simulink model "PubIfFusionRFM_MDL"  (R2020b)
settings: Solver=FixedStepAuto  StartTime=0.0  StopTime=Inf  RelTol=1e-3
PostLoadFcn:
  | if any(exist('dsrtsu_mdlpostloadfcn', 'file') ~= 0), dsrtsu_mdlpostloadfcn('Execute', bdroot); end
InitFcn:
  | , if any(exist('dsmpb_private', 'file') ~= 0), dsmpb_private('dsmpb_mdlclblib', 'Init', bdroot); end,
model workspace (MAT data in the model file):
  EQ4COM_BrkPedalSts = Simulink.Signal
  EQ4COM_BrkPedalSts.DataType = 'auto'
  EQ4COM_BrkPedalSts.Dimensions = -1
  EQ4COM_BrkPedalSts.DimensionsMode = 'auto'
  EQ4COM_BrkPedalSts.Complexity = 'auto'
  EQ4COM_BrkPedalSts.SampleTime = -1
  EQ4COM_BrkPedalSts.SamplingMode = 'auto'
  EQ4COM_ESP_MasterCylBrkPress = Simulink.Signal
  EQ4COM_ESP_MasterCylBrkPress.DataType = 'auto'
  EQ4COM_ESP_MasterCylBrkPress.Dimensions = -1
  EQ4COM_ESP_MasterCylBrkPress.DimensionsMode = 'auto'
  EQ4COM_ESP_MasterCylBrkPress.Complexity = 'auto'
  EQ4COM_ESP_MasterCylBrkPress.SampleTime = -1
  EQ4COM_ESP_MasterCylBrkPress.SamplingMode = 'auto'
  EQ4COM_SteerWheelAng = Simulink.Signal
  EQ4COM_SteerWheelAng.DataType = 'auto'
  EQ4COM_SteerWheelAng.Dimensions = -1
  EQ4COM_SteerWheelAng.DimensionsMode = 'auto'
  EQ4COM_SteerWheelAng.Complexity = 'auto'
  EQ4COM_SteerWheelAng.SampleTime = -1
  EQ4COM_SteerWheelAng.SamplingMode = 'auto'
  EQ4COM_SteerWheelAngSign = Simulink.Signal
  EQ4COM_SteerWheelAngSign.DataType = 'auto'
  EQ4COM_SteerWheelAngSign.Dimensions = -1
  EQ4COM_SteerWheelAngSign.DimensionsMode = 'auto'
  EQ4COM_SteerWheelAngSign.Complexity = 'auto'
  EQ4COM_SteerWheelAngSign.SampleTime = -1
  EQ4COM_SteerWheelAngSign.SamplingMode = 'auto'
  EQ4COM_VehLatAccel = Simulink.Signal
  EQ4COM_VehLatAccel.DataType = 'auto'
  EQ4COM_VehLatAccel.Dimensions = -1
  EQ4COM_VehLatAccel.DimensionsMode = 'auto'
  EQ4COM_VehLatAccel.Complexity = 'auto'
  EQ4COM_VehLatAccel.SampleTime = -1
  EQ4COM_VehLatAccel.SamplingMode = 'auto'
  EQ4COM_VehLgtAccel = Simulink.Signal
  EQ4COM_VehLgtAccel.DataType = 'auto'
  EQ4COM_VehLgtAccel.Dimensions = -1
  EQ4COM_VehLgtAccel.DimensionsMode = 'auto'
  EQ4COM_VehLgtAccel.Complexity = 'auto'
  EQ4COM_VehLgtAccel.SampleTime = -1
  EQ4COM_VehLgtAccel.SamplingMode = 'auto'
  EQ4COM_VehSpd = Simulink.Signal
  EQ4COM_VehSpd.DataType = 'auto'
  EQ4COM_VehSpd.Dimensions = -1
  EQ4COM_VehSpd.DimensionsMode = 'auto'
  EQ4COM_VehSpd.Complexity = 'auto'
  EQ4COM_VehSpd.SampleTime = -1
  EQ4COM_VehSpd.SamplingMode = 'auto'
  EQ4COM_VehYawRate = Simulink.Signal
  EQ4COM_VehYawRate.DataType = 'auto'
  EQ4COM_VehYawRate.Dimensions = -1
  EQ4COM_VehYawRate.DimensionsMode = 'auto'
  EQ4COM_VehYawRate.Complexity = 'auto'
  EQ4COM_VehYawRate.SampleTime = -1
  EQ4COM_VehYawRate.SamplingMode = 'auto'
PreSaveFcn:
  | , if any(exist('dsmpb_private', 'file') ~= 0), dsmpb_private('dsmpb_mdlclblib', 'PreSave', bdroot); end,
CloseFcn:
  | , if any(exist('dsmpb_private', 'file') ~= 0), dsmpb_private('dsmpb_mdlclblib', 'Close', bdroot); end,
settings Model: DataDictionary=HWA_DDs.sldd  RTICANMMDATA=struct('GeneralSetupData',struct('modelroot','C:\Users\GW00133806\Desktop\ADAS_Store\Project\V61_Autobox_Noa\Fusion\fusRoad','generalsettings',struct('filesettings',struct('destfolder',struct('Name','RTICANMM_FILES','Check',1),'buildfolder',struct('Name','.','Check',1),'AbsDestfolder',struct('Name','C:\Users\GW00133806\Desktop\ADAS_Store\Project\V61_Autobox_Noa\Fusion\fusRoad\RTICANMM_FILES'),'AbsBuildfolder',struct('Name','C:\Users\GW00133806\Desktop\ADAS_Store\Project\V61_Autobox_Noa\Fusion\fusRoad'))),'options',struct('addpaths',1,'rmpaths',1,'addtrcexclusion',false,'cannavigator',struct('checkmonitoring',0),'show_usrtrc',0,'use_usrtrc',0),'advanced',struct('options',ones(1,100)),'MPSetup',{{}},'RTI',struct('Type','DSRT','Ver','4.2','Date','02-Nov-2019'),'modelname','PubIfFusionRFM_MDL','block','PubIfFusionRFM_MDL'))  DSRTSU_INTERNAL_RTIFPGA=150  Creator=GW00180895  LastModifiedBy=GW00133806
settings OptimizationCC: BlockReduction=off  ConditionallyExecuteInputs=off  OptimizeBlockIOStorage=off  BufferReuse=off
settings DebuggingCC: TasksWithSamePriorityMsg=none
settings HardwareCC: ProdBitPerPointer=32  ProdBitPerSizeT=32  ProdBitPerPtrDiffT=32  ProdLargestAtomicInteger=Integer  ProdWordSize=32  ProdHWDeviceType=Custom Processor->Custom
settings ModelReferenceCC: EnableParallelModelReferenceBuilds=on  ModelReferenceNumInstancesAllowed=Single  SupportModelReferenceSimTargetCustomCode=on
settings SFSimCC: SimParseCustomCode=off  MATLABDynamicMemAlloc=off
settings SFSimCC: SimUserSources=|
  | FusionApi.c
  | HWAapi.c
  | HWA_R.c
  | HWAafRoadArithm.c
  | HWABoundary.c
  | HWABoundaryLinePredicted.c
  | HWALineFusion.c
  | HWAObejctManage.c
  | HWARoadLayout.c
  | HWARoadPreprocess.c
  | HWARoadSceneRecognition.c
  | HWASpeedLimit.c
  | HWAOutputSendCallback.c
settings SFSimCC: SimUserIncludeDirs=|
  | .\src\HWA_Road\include
  | .\src\HWA_Road\include\HWAMsg
  | .\src\HWA_Road\include\HWAPack
  | .\src\HWA_Road\include\HWAApi
  | .\src\HWA_Road\source
  | .\src\HWA_Road\source\Road
  | .\src\HWA_Road_Api
  | .\src\HWA_Road_Api\autosar_swc_infofusion_autosar_rtw
  | .\src
settings RTWCC: Description=dSPACE Run-Time Target (for VEOS on Windows and ConfigurationDesk)  SystemTargetFile=dsrt.tlc  GenCodeOnly=on  MakeCommand=make_dsrt  TemplateMakefile=dsrt_default_tmf  RTWVerbose=off  RTWUseSimCustomCode=on
settings RTWCC: CustomInclude=|
  | .\src\HWA_Road\include
  | .\src\HWA_Road\include\HWAMsg
  | .\src\HWA_Road\include\HWAPack
  | .\src\HWA_Road\include\HWAApi
  | .\src\HWA_Road\source
  | .\src\HWA_Road\source\Road
  | .\src\HWA_Road_Api
  | .\src\HWA_Road_Api\autosar_swc_infofusion_autosar_rtw
  | .\src
settings RTWCC: CustomSource=|
  | FusionApi.c
  | HWAapi.c
  | HWA_R.c
  | HWAafRoadArithm.c
  | HWABoundary.c
  | HWABoundaryLinePredicted.c
  | HWALineFusion.c
  | HWAObejctManage.c
  | HWARoadLayout.c
  | HWARoadPreprocess.c
  | HWARoadSceneRecognition.c
  | HWASpeedLimit.c
  | HWAOutputSendCallback.c
settings STFCustomTargetCC: TargetLangStandard=C99 (ISO)  ParMdlRefBuildCompliant=on  ConcurrentExecutionCompliant=off  CPPClassGenCompliant=off  GRTInterface=off  SystemTargetFile=dsrt.tlc
settings GRTTargetCC: CompOptLevelCompliant=off  ConcurrentExecutionCompliant=off  CombineOutputUpdateFcns=off  MatFileLogging=off  CPPClassGenCompliant=off  UseToolchainInfoCompliant=off

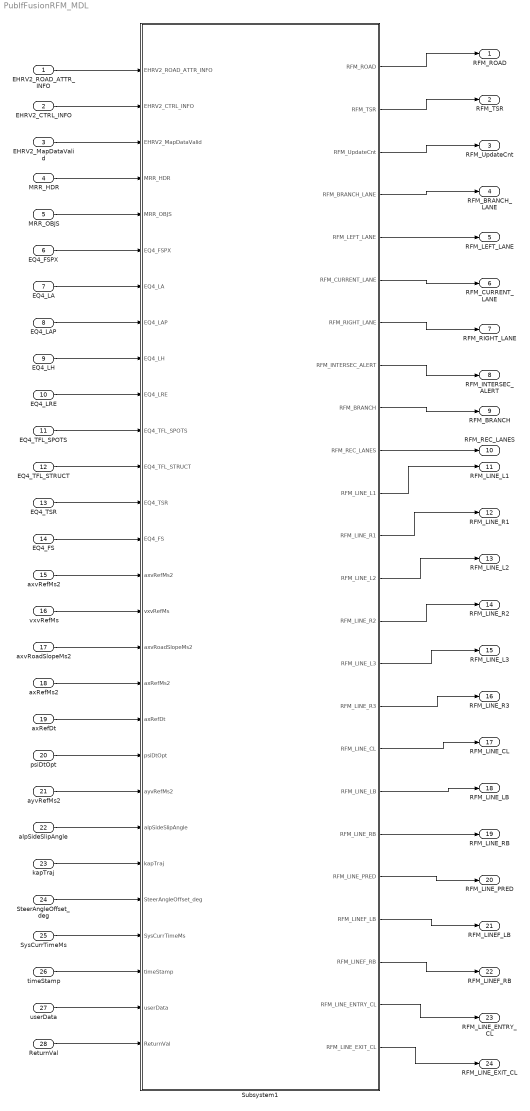
== system PubIfFusionRFM_MDL ==
  EHRV2_ROAD_ATTR_INFO : Inport  OutDataTypeStr=Bus: EHRV2_ROAD_ATTR_INFO_BUS  PortDimensions=1  BusOutputAsStruct=on
  EHRV2_CTRL_INFO : Inport  Port=2  OutDataTypeStr=Bus: EHRV2_CTRL_INFO_BUS  PortDimensions=1  BusOutputAsStruct=on
  EHRV2_MapDataValid : Inport  Port=3  OutDataTypeStr=uint8  PortDimensions=1  BusOutputAsStruct=on
  MRR_HDR : Inport  Port=4  OutDataTypeStr=Bus: MRR_HDR_BUS  PortDimensions=1  BusOutputAsStruct=on
  MRR_OBJS : Inport  Port=5  OutDataTypeStr=Bus: MRR_OBJ_BUS  PortDimensions=32  BusOutputAsStruct=on
  EQ4_FSPX : Inport  Port=6  OutDataTypeStr=Bus: EQ4_FSPX_BUS  PortDimensions=1  BusOutputAsStruct=on
  EQ4_LA : Inport  Port=7  OutDataTypeStr=Bus: EQ4_LA_BUS  PortDimensions=1  BusOutputAsStruct=on
  EQ4_LAP : Inport  Port=8  OutDataTypeStr=Bus: EQ4_LAP_BUS  PortDimensions=1  BusOutputAsStruct=on
  EQ4_LH : Inport  Port=9  OutDataTypeStr=Bus: EQ4_LH_BUS  PortDimensions=1  BusOutputAsStruct=on
  EQ4_LRE : Inport  Port=10  OutDataTypeStr=Bus: EQ4_LRE_BUS  PortDimensions=1  BusOutputAsStruct=on
  EQ4_TFL_SPOTS : Inport  Port=11  OutDataTypeStr=Bus: EQ4_TFL_SPOTS_BUS  PortDimensions=1  BusOutputAsStruct=on
  EQ4_TFL_STRUCT : Inport  Port=12  OutDataTypeStr=Bus: EQ4_TFL_STRUCT_BUS  PortDimensions=1  BusOutputAsStruct=on
  EQ4_TSR : Inport  Port=13  OutDataTypeStr=Bus: EQ4_TSR_BUS  PortDimensions=1  BusOutputAsStruct=on
  EQ4_FS : Inport  Port=14  OutDataTypeStr=Bus: EQ4_FS_BUS  PortDimensions=1  BusOutputAsStruct=on
  axvRefMs2 : Inport  Port=15  OutDataTypeStr=single  PortDimensions=1  BusOutputAsStruct=on
  vxvRefMs : Inport  Port=16  OutDataTypeStr=single  PortDimensions=1  BusOutputAsStruct=on
  axvRoadSlopeMs2 : Inport  Port=17  OutDataTypeStr=single  PortDimensions=1  BusOutputAsStruct=on
  axRefMs2 : Inport  Port=18  OutDataTypeStr=single  PortDimensions=1  BusOutputAsStruct=on
  axRefDt : Inport  Port=19  OutDataTypeStr=single  PortDimensions=1  BusOutputAsStruct=on
  psiDtOpt : Inport  Port=20  OutDataTypeStr=single  PortDimensions=1  BusOutputAsStruct=on
  ayvRefMs2 : Inport  Port=21  OutDataTypeStr=single  PortDimensions=1  BusOutputAsStruct=on
  alpSideSlipAngle : Inport  Port=22  OutDataTypeStr=single  PortDimensions=1  BusOutputAsStruct=on
  kapTraj : Inport  Port=23  OutDataTypeStr=single  PortDimensions=1  BusOutputAsStruct=on
  SteerAngleOffset_deg : Inport  Port=24  OutDataTypeStr=single  PortDimensions=1  BusOutputAsStruct=on
  SysCurrTimeMs : Inport  Port=25  OutDataTypeStr=uint32  PortDimensions=1  BusOutputAsStruct=on
  timeStamp : Inport  Port=26  OutDataTypeStr=Bus: StbM_TimeStampExtendedType  PortDimensions=1  BusOutputAsStruct=on
  userData : Inport  Port=27  OutDataTypeStr=Bus: StbM_UserDataType  PortDimensions=1  BusOutputAsStruct=on
  ReturnVal : Inport  Port=28  OutDataTypeStr=uint8  PortDimensions=1  BusOutputAsStruct=on
  Subsystem1 : Subsystem
  RFM_ROAD : Outport  OutDataTypeStr=Bus: RFM_ROAD_BUS  BusOutputAsStruct=on
  RFM_TSR : Outport  Port=2  OutDataTypeStr=Bus: RFM_TSR_BUS  PortDimensions=1  BusOutputAsStruct=on
  RFM_UpdateCnt : Outport  Port=3  OutDataTypeStr=uint32  PortDimensions=1  BusOutputAsStruct=on
  RFM_BRANCH_LANE : Outport  Port=4  OutDataTypeStr=Bus: RFM_LANE_BUS  PortDimensions=1  BusOutputAsStruct=on
  RFM_LEFT_LANE : Outport  Port=5  OutDataTypeStr=Bus: RFM_LANE_BUS  PortDimensions=1  BusOutputAsStruct=on
  RFM_CURRENT_LANE : Outport  Port=6  OutDataTypeStr=Bus: RFM_LANE_BUS  PortDimensions=1  BusOutputAsStruct=on
  RFM_RIGHT_LANE : Outport  Port=7  OutDataTypeStr=Bus: RFM_LANE_BUS  PortDimensions=1  BusOutputAsStruct=on
  RFM_INTERSEC_ALERT : Outport  Port=8  OutDataTypeStr=Bus: RFM_INTERSEC_ALERT_BUS  PortDimensions=1  BusOutputAsStruct=on
  RFM_BRANCH : Outport  Port=9  OutDataTypeStr=Bus: RFM_BRANCH_BUS  PortDimensions=1  BusOutputAsStruct=on
  RFM_REC_LANES : Outport  Port=10  OutDataTypeStr=Bus: RFM_REC_LANES_BUS  PortDimensions=1  BusOutputAsStruct=on
  RFM_LINE_L1 : Outport  Port=11  OutDataTypeStr=Bus: RFM_LINE_BUS  PortDimensions=1  BusOutputAsStruct=on
  RFM_LINE_R1 : Outport  Port=12  OutDataTypeStr=Bus: RFM_LINE_BUS  PortDimensions=1  BusOutputAsStruct=on
  RFM_LINE_L2 : Outport  Port=13  OutDataTypeStr=Bus: RFM_LINE_BUS  PortDimensions=1  BusOutputAsStruct=on
  RFM_LINE_R2 : Outport  Port=14  OutDataTypeStr=Bus: RFM_LINE_BUS  PortDimensions=1  BusOutputAsStruct=on
  RFM_LINE_L3 : Outport  Port=15  OutDataTypeStr=Bus: RFM_LINE_BUS  PortDimensions=1  BusOutputAsStruct=on
  RFM_LINE_R3 : Outport  Port=16  OutDataTypeStr=Bus: RFM_LINE_BUS  PortDimensions=1  BusOutputAsStruct=on
  RFM_LINE_CL : Outport  Port=17  OutDataTypeStr=Bus: RFM_LINE_BUS  PortDimensions=1  BusOutputAsStruct=on
  RFM_LINE_LB : Outport  Port=18  OutDataTypeStr=Bus: RFM_LINE_BUS  PortDimensions=1  BusOutputAsStruct=on
  RFM_LINE_RB : Outport  Port=19  OutDataTypeStr=Bus: RFM_LINE_BUS  PortDimensions=1  BusOutputAsStruct=on
  RFM_LINE_PRED : Outport  Port=20  OutDataTypeStr=Bus: RFM_LINE_BUS  PortDimensions=1  BusOutputAsStruct=on
  RFM_LINEF_LB : Outport  Port=21  OutDataTypeStr=Bus: RFM_LINE_BUS  PortDimensions=1  BusOutputAsStruct=on
  RFM_LINEF_RB : Outport  Port=22  OutDataTypeStr=Bus: RFM_LINE_BUS  PortDimensions=1  BusOutputAsStruct=on
  RFM_LINE_ENTRY_CL : Outport  Port=23  OutDataTypeStr=Bus: RFM_LINE_BUS  PortDimensions=1  BusOutputAsStruct=on
  RFM_LINE_EXIT_CL : Outport  Port=24  OutDataTypeStr=Bus: RFM_LINE_BUS  PortDimensions=1  BusOutputAsStruct=on
  wires:
  EHRV2_ROAD_ATTR_INFO/1 -> Subsystem1/1(EHRV2_ROAD_ATTR_INFO)
  EHRV2_CTRL_INFO/1 -> Subsystem1/2(EHRV2_CTRL_INFO)
  EHRV2_MapDataValid/1 -> Subsystem1/3(EHRV2_MapDataValid)
  MRR_HDR/1 -> Subsystem1/4(MRR_HDR)
  MRR_OBJS/1 -> Subsystem1/5(MRR_OBJS)
  EQ4_FSPX/1 -> Subsystem1/6(EQ4_FSPX)
  EQ4_LA/1 -> Subsystem1/7(EQ4_LA)
  EQ4_LAP/1 -> Subsystem1/8(EQ4_LAP)
  EQ4_LH/1 -> Subsystem1/9(EQ4_LH)
  EQ4_LRE/1 -> Subsystem1/10(EQ4_LRE)
  EQ4_TFL_SPOTS/1 -> Subsystem1/11(EQ4_TFL_SPOTS)
  EQ4_TFL_STRUCT/1 -> Subsystem1/12(EQ4_TFL_STRUCT)
  EQ4_TSR/1 -> Subsystem1/13(EQ4_TSR)
  EQ4_FS/1 -> Subsystem1/14(EQ4_FS)
  axvRefMs2/1 -> Subsystem1/15(axvRefMs2)
  vxvRefMs/1 -> Subsystem1/16(vxvRefMs)
  axvRoadSlopeMs2/1 -> Subsystem1/17(axvRoadSlopeMs2)
  axRefMs2/1 -> Subsystem1/18(axRefMs2)
  axRefDt/1 -> Subsystem1/19(axRefDt)
  psiDtOpt/1 -> Subsystem1/20(psiDtOpt)
  ayvRefMs2/1 -> Subsystem1/21(ayvRefMs2)
  alpSideSlipAngle/1 -> Subsystem1/22(alpSideSlipAngle)
  kapTraj/1 -> Subsystem1/23(kapTraj)
  SteerAngleOffset_deg/1 -> Subsystem1/24(SteerAngleOffset_deg)
  SysCurrTimeMs/1 -> Subsystem1/25(SysCurrTimeMs)
  timeStamp/1 -> Subsystem1/26(timeStamp)
  userData/1 -> Subsystem1/27(userData)
  ReturnVal/1 -> Subsystem1/28(ReturnVal)
  Subsystem1/1(RFM_ROAD) -> RFM_ROAD/1
  Subsystem1/2(RFM_TSR) -> RFM_TSR/1
  Subsystem1/3(RFM_UpdateCnt) -> RFM_UpdateCnt/1
  Subsystem1/4(RFM_BRANCH_LANE) -> RFM_BRANCH_LANE/1
  Subsystem1/5(RFM_LEFT_LANE) -> RFM_LEFT_LANE/1
  Subsystem1/6(RFM_CURRENT_LANE) -> RFM_CURRENT_LANE/1
  Subsystem1/7(RFM_RIGHT_LANE) -> RFM_RIGHT_LANE/1
  Subsystem1/8(RFM_INTERSEC_ALERT) -> RFM_INTERSEC_ALERT/1
  Subsystem1/10(RFM_REC_LANES) -> RFM_REC_LANES/1
  Subsystem1/11(RFM_LINE_L1) -> RFM_LINE_L1/1
  Subsystem1/12(RFM_LINE_R1) -> RFM_LINE_R1/1
  Subsystem1/13(RFM_LINE_L2) -> RFM_LINE_L2/1
  Subsystem1/14(RFM_LINE_R2) -> RFM_LINE_R2/1
  Subsystem1/15(RFM_LINE_L3) -> RFM_LINE_L3/1
  Subsystem1/16(RFM_LINE_R3) -> RFM_LINE_R3/1
  Subsystem1/17(RFM_LINE_CL) -> RFM_LINE_CL/1
  Subsystem1/18(RFM_LINE_LB) -> RFM_LINE_LB/1
  Subsystem1/19(RFM_LINE_RB) -> RFM_LINE_RB/1
  Subsystem1/20(RFM_LINE_PRED) -> RFM_LINE_PRED/1
  Subsystem1/21(RFM_LINEF_LB) -> RFM_LINEF_LB/1
  Subsystem1/22(RFM_LINEF_RB) -> RFM_LINEF_RB/1
  Subsystem1/23(RFM_LINE_ENTRY_CL) -> RFM_LINE_ENTRY_CL/1
  Subsystem1/24(RFM_LINE_EXIT_CL) -> RFM_LINE_EXIT_CL/1
  Subsystem1/9(RFM_BRANCH) -> RFM_BRANCH/1

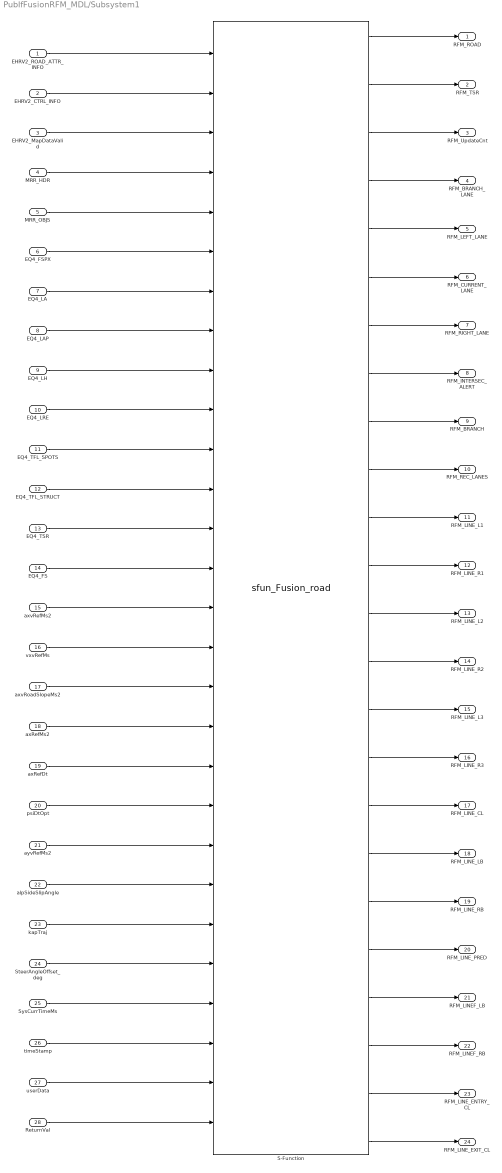
== system PubIfFusionRFM_MDL/Subsystem1 ==
  EHRV2_ROAD_ATTR_INFO : Inport  OutDataTypeStr=Bus: EHRV2_ROAD_ATTR_INFO_BUS  PortDimensions=1  BusOutputAsStruct=on
  EHRV2_CTRL_INFO : Inport  Port=2  OutDataTypeStr=Bus: EHRV2_CTRL_INFO_BUS  PortDimensions=1  BusOutputAsStruct=on
  EHRV2_MapDataValid : Inport  Port=3  OutDataTypeStr=uint8  PortDimensions=1  BusOutputAsStruct=on
  MRR_HDR : Inport  Port=4  OutDataTypeStr=Bus: MRR_HDR_BUS  PortDimensions=1  BusOutputAsStruct=on
  MRR_OBJS : Inport  Port=5  OutDataTypeStr=Bus: MRR_OBJ_BUS  PortDimensions=32  BusOutputAsStruct=on
  EQ4_FSPX : Inport  Port=6  OutDataTypeStr=Bus: EQ4_FSPX_BUS  PortDimensions=1  BusOutputAsStruct=on
  EQ4_LA : Inport  Port=7  OutDataTypeStr=Bus: EQ4_LA_BUS  PortDimensions=1  BusOutputAsStruct=on
  EQ4_LAP : Inport  Port=8  OutDataTypeStr=Bus: EQ4_LAP_BUS  PortDimensions=1  BusOutputAsStruct=on
  EQ4_LH : Inport  Port=9  OutDataTypeStr=Bus: EQ4_LH_BUS  PortDimensions=1  BusOutputAsStruct=on
  EQ4_LRE : Inport  Port=10  OutDataTypeStr=Bus: EQ4_LRE_BUS  PortDimensions=1  BusOutputAsStruct=on
  EQ4_TFL_SPOTS : Inport  Port=11  OutDataTypeStr=Bus: EQ4_TFL_SPOTS_BUS  PortDimensions=1  BusOutputAsStruct=on
  EQ4_TFL_STRUCT : Inport  Port=12  OutDataTypeStr=Bus: EQ4_TFL_STRUCT_BUS  PortDimensions=1  BusOutputAsStruct=on
  EQ4_TSR : Inport  Port=13  OutDataTypeStr=Bus: EQ4_TSR_BUS  PortDimensions=1  BusOutputAsStruct=on
  EQ4_FS : Inport  Port=14  OutDataTypeStr=Bus: EQ4_FS_BUS  PortDimensions=1  BusOutputAsStruct=on
  axvRefMs2 : Inport  Port=15  OutDataTypeStr=single  PortDimensions=1  BusOutputAsStruct=on
  vxvRefMs : Inport  Port=16  OutDataTypeStr=single  PortDimensions=1  BusOutputAsStruct=on
  axvRoadSlopeMs2 : Inport  Port=17  OutDataTypeStr=single  PortDimensions=1  BusOutputAsStruct=on
  axRefMs2 : Inport  Port=18  OutDataTypeStr=single  PortDimensions=1  BusOutputAsStruct=on
  axRefDt : Inport  Port=19  OutDataTypeStr=single  PortDimensions=1  BusOutputAsStruct=on
  psiDtOpt : Inport  Port=20  OutDataTypeStr=single  PortDimensions=1  BusOutputAsStruct=on
  ayvRefMs2 : Inport  Port=21  OutDataTypeStr=single  PortDimensions=1  BusOutputAsStruct=on
  alpSideSlipAngle : Inport  Port=22  OutDataTypeStr=single  PortDimensions=1  BusOutputAsStruct=on
  kapTraj : Inport  Port=23  OutDataTypeStr=single  PortDimensions=1  BusOutputAsStruct=on
  SteerAngleOffset_deg : Inport  Port=24  OutDataTypeStr=single  PortDimensions=1  BusOutputAsStruct=on
  SysCurrTimeMs : Inport  Port=25  OutDataTypeStr=uint32  PortDimensions=1  BusOutputAsStruct=on
  timeStamp : Inport  Port=26  OutDataTypeStr=Bus: StbM_TimeStampExtendedType  PortDimensions=1  BusOutputAsStruct=on
  userData : Inport  Port=27  OutDataTypeStr=Bus: StbM_UserDataType  PortDimensions=1  BusOutputAsStruct=on
  ReturnVal : Inport  Port=28  OutDataTypeStr=uint8  PortDimensions=1  BusOutputAsStruct=on
  S-Function : S-Function  FunctionName=sfun_Fusion_road  SFunctionDeploymentMode=off  EnableBusSupport=off
  RFM_ROAD : Outport  OutDataTypeStr=Bus: RFM_ROAD_BUS  BusOutputAsStruct=on
  RFM_TSR : Outport  Port=2  OutDataTypeStr=Bus: RFM_TSR_BUS  PortDimensions=1  BusOutputAsStruct=on
  RFM_UpdateCnt : Outport  Port=3  OutDataTypeStr=uint32  PortDimensions=1  BusOutputAsStruct=on
  RFM_BRANCH_LANE : Outport  Port=4  OutDataTypeStr=Bus: RFM_LANE_BUS  PortDimensions=1  BusOutputAsStruct=on
  RFM_LEFT_LANE : Outport  Port=5  OutDataTypeStr=Bus: RFM_LANE_BUS  PortDimensions=1  BusOutputAsStruct=on
  RFM_CURRENT_LANE : Outport  Port=6  OutDataTypeStr=Bus: RFM_LANE_BUS  PortDimensions=1  BusOutputAsStruct=on
  RFM_RIGHT_LANE : Outport  Port=7  OutDataTypeStr=Bus: RFM_LANE_BUS  PortDimensions=1  BusOutputAsStruct=on
  RFM_INTERSEC_ALERT : Outport  Port=8  OutDataTypeStr=Bus: RFM_INTERSEC_ALERT_BUS  PortDimensions=1  BusOutputAsStruct=on
  RFM_BRANCH : Outport  Port=9  OutDataTypeStr=Bus: RFM_BRANCH_BUS  PortDimensions=1  BusOutputAsStruct=on
  RFM_REC_LANES : Outport  Port=10  OutDataTypeStr=Bus: RFM_REC_LANES_BUS  PortDimensions=1  BusOutputAsStruct=on
  RFM_LINE_L1 : Outport  Port=11  OutDataTypeStr=Bus: RFM_LINE_BUS  PortDimensions=1  BusOutputAsStruct=on
  RFM_LINE_R1 : Outport  Port=12  OutDataTypeStr=Bus: RFM_LINE_BUS  PortDimensions=1  BusOutputAsStruct=on
  RFM_LINE_L2 : Outport  Port=13  OutDataTypeStr=Bus: RFM_LINE_BUS  PortDimensions=1  BusOutputAsStruct=on
  RFM_LINE_R2 : Outport  Port=14  OutDataTypeStr=Bus: RFM_LINE_BUS  PortDimensions=1  BusOutputAsStruct=on
  RFM_LINE_L3 : Outport  Port=15  OutDataTypeStr=Bus: RFM_LINE_BUS  PortDimensions=1  BusOutputAsStruct=on
  RFM_LINE_R3 : Outport  Port=16  OutDataTypeStr=Bus: RFM_LINE_BUS  PortDimensions=1  BusOutputAsStruct=on
  RFM_LINE_CL : Outport  Port=17  OutDataTypeStr=Bus: RFM_LINE_BUS  PortDimensions=1  BusOutputAsStruct=on
  RFM_LINE_LB : Outport  Port=18  OutDataTypeStr=Bus: RFM_LINE_BUS  PortDimensions=1  BusOutputAsStruct=on
  RFM_LINE_RB : Outport  Port=19  OutDataTypeStr=Bus: RFM_LINE_BUS  PortDimensions=1  BusOutputAsStruct=on
  RFM_LINE_PRED : Outport  Port=20  OutDataTypeStr=Bus: RFM_LINE_BUS  PortDimensions=1  BusOutputAsStruct=on
  RFM_LINEF_LB : Outport  Port=21  OutDataTypeStr=Bus: RFM_LINE_BUS  PortDimensions=1  BusOutputAsStruct=on
  RFM_LINEF_RB : Outport  Port=22  OutDataTypeStr=Bus: RFM_LINE_BUS  PortDimensions=1  BusOutputAsStruct=on
  RFM_LINE_ENTRY_CL : Outport  Port=23  OutDataTypeStr=Bus: RFM_LINE_BUS  PortDimensions=1  BusOutputAsStruct=on
  RFM_LINE_EXIT_CL : Outport  Port=24  OutDataTypeStr=Bus: RFM_LINE_BUS  PortDimensions=1  BusOutputAsStruct=on
  wires:
  EHRV2_ROAD_ATTR_INFO/1 -> S-Function/1
  EHRV2_CTRL_INFO/1 -> S-Function/2
  EHRV2_MapDataValid/1 -> S-Function/3
  MRR_HDR/1 -> S-Function/4
  MRR_OBJS/1 -> S-Function/5
  EQ4_FSPX/1 -> S-Function/6
  EQ4_LA/1 -> S-Function/7
  EQ4_LAP/1 -> S-Function/8
  EQ4_LH/1 -> S-Function/9
  EQ4_LRE/1 -> S-Function/10
  EQ4_TFL_SPOTS/1 -> S-Function/11
  EQ4_TFL_STRUCT/1 -> S-Function/12
  EQ4_TSR/1 -> S-Function/13
  EQ4_FS/1 -> S-Function/14
  axvRefMs2/1 -> S-Function/15
  vxvRefMs/1 -> S-Function/16
  axvRoadSlopeMs2/1 -> S-Function/17
  axRefMs2/1 -> S-Function/18
  axRefDt/1 -> S-Function/19
  psiDtOpt/1 -> S-Function/20
  ayvRefMs2/1 -> S-Function/21
  alpSideSlipAngle/1 -> S-Function/22
  kapTraj/1 -> S-Function/23
  SteerAngleOffset_deg/1 -> S-Function/24
  SysCurrTimeMs/1 -> S-Function/25
  timeStamp/1 -> S-Function/26
  userData/1 -> S-Function/27
  ReturnVal/1 -> S-Function/28
  S-Function/1 -> RFM_ROAD/1
  S-Function/2 -> RFM_TSR/1
  S-Function/3 -> RFM_UpdateCnt/1
  S-Function/4 -> RFM_BRANCH_LANE/1
  S-Function/5 -> RFM_LEFT_LANE/1
  S-Function/6 -> RFM_CURRENT_LANE/1
  S-Function/7 -> RFM_RIGHT_LANE/1
  S-Function/8 -> RFM_INTERSEC_ALERT/1
  S-Function/10 -> RFM_REC_LANES/1
  S-Function/11 -> RFM_LINE_L1/1
  S-Function/12 -> RFM_LINE_R1/1
  S-Function/13 -> RFM_LINE_L2/1
  S-Function/14 -> RFM_LINE_R2/1
  S-Function/15 -> RFM_LINE_L3/1
  S-Function/16 -> RFM_LINE_R3/1
  S-Function/17 -> RFM_LINE_CL/1
  S-Function/18 -> RFM_LINE_LB/1
  S-Function/19 -> RFM_LINE_RB/1
  S-Function/20 -> RFM_LINE_PRED/1
  S-Function/21 -> RFM_LINEF_LB/1
  S-Function/22 -> RFM_LINEF_RB/1
  S-Function/23 -> RFM_LINE_ENTRY_CL/1
  S-Function/24 -> RFM_LINE_EXIT_CL/1
  S-Function/9 -> RFM_BRANCH/1
